simulink model "gm_untitled"  (R2020b)
settings: Solver=VariableStepAuto  StartTime=0.0  StopTime=0.001  RelTol=1e-3
undefined symbols (not defined in the file or in its folder): dspDeleteFVToolLinkFromMask, gcbh
libraries: simulink x1, dsparch4 x1
settings Model: Creator=pablo  LastModifiedBy=pablo
settings OptimizationCC: BlockReduction=off  ConditionallyExecuteInputs=off
settings DebuggingCC: InheritedTsInSrcMsg=none

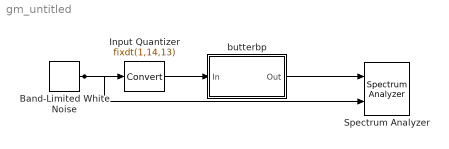
== system gm_untitled ==
  Band-Limited White Noise : simulink/Sources/Band-Limited White Noise  Cov=[0.1]  Ts=0.1  seed=[23341]
  Input Quantizer : DataTypeConversion  OutDataTypeStr=fixdt(1,14,13)  RndMeth=Round  SaturateOnIntegerOverflow=on
  Spectrum Analyzer : SpectrumAnalyzer  NumInputPorts=2
  butterbp : Subsystem
  wires:
  Band-Limited White Noise/1 -> Input Quantizer/1, Spectrum Analyzer/2
  butterbp/1(Out) -> Spectrum Analyzer/1
  Input Quantizer/1 -> butterbp/1(In)

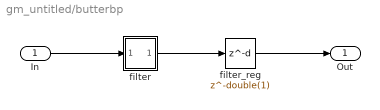
== system gm_untitled/butterbp ==
  In : Inport  OutDataTypeStr=fixdt(1, 14, 13)  PortDimensions=1  SampleTime=0.1
  filter : Subsystem  LoadFcn=dspDeleteFVToolLinkFromMask(gcbh);
      settings: DeleteFcn=dspLinkFVTool2Mask(gcbh,'close')  ModelCloseFcn=dspLinkFVTool2Mask(gcbh,'close')  PreSaveFcn=dspUnlinkFVToolFromMask(gcbh);  PostSaveFcn=dspRestoreLinkFVTool2Mask(gcbh);  CloseFcn=dspLinkFVTool2Mask(gcbh,'close')
      settings: CopyFcn=|
      | ud = get_param(gcbh,'UserData');
      | if isfield(ud,'fvtool')
      |   ud = rmfield(ud,'fvtool');
      |   set_param(gcbh,'UserData',ud);
      | end
      | clear ud
  filter_reg : Delay  DelayLength=double(1)  InitialCondition=0  SampleTime=0.1
  Out : Outport
  wires:
  In/1 -> filter/1(In1)
  filter_reg/1 -> Out/1
  filter/1(Out1) -> filter_reg/1

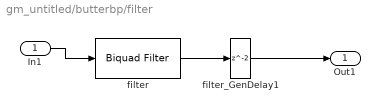
== system gm_untitled/butterbp/filter ==
  In1 : Inport
  filter : dsparch4/Biquad Filter  FilterSource=Dialog parameters  CoeffSource=Specify via dialog  FilterObject=BQF  IIRFiltStruct=Direct form II  BiQuadCoeffs=[1 0 -1 1 -1.60137133706940249 0.992507630825395504;1 0 -1 1 -1.62252630353837413 0.992689665899144646;1 0 -1 1 -1.59926077751646867 0.982133309763404405;1 0 -1 1 -1.60806350104833395 0.982313500850860999]  ScaleValues=[0.00967072626983317592;0.00967072626983317592;0.0096206923413178231;0.0096206923413178231;1]  IC=0  ICnum=0  ICden=0  a0Flag=Warning  optimizeScaleValues=on  ScaleValueMode=Specify via input port (g)  InputProcessing=Columns as channels (frame based)  roundingMode=Convergent  overflowMode=off  stageInputMode=Binary point scaling  stageInputWordLength=16  stageInputFracLength=16  stageOutputMode=Binary point scaling  stageOutputWordLength=16  stageOutputFracLength=11  firstCoeffMode=Binary point scaling  firstCoeffWordLength=16  firstCoeffFracLength=14  scaleValueFracLength=21  prodOutputMode=Binary point scaling  prodOutputWordLength=32  prodOutputFracLength=29  denProdOutputFracLength=29  accumMode=Binary point scaling  accumWordLength=40  accumFracLength=29  denAccumFracLength=29  memoryMode=Binary point scaling  memoryWordLength=16  memoryFracLength=15  secondMemoryFracLength=15  outputMode=Binary point scaling  outputWordLength=18  outputFracLength=13
  filter_GenDelay1 : Delay
  Out1 : Outport
  wires:
  In1/1 -> filter/1
  filter/1 -> filter_GenDelay1/1
  filter_GenDelay1/1 -> Out1/1
